simulink model "simulation_ENMPC"  (R2018a)
settings: Solver=ode15s  StartTime=0.0  StopTime=T  RelTol=1e-3
values from neighbouring files (symbols this model uses):
  c = G\Uf    [main_approx_NMPC.m]
  x0 = xk(:)    [find_optimal_NMPC.m]    (also in main_approx_NMPC.m = MPC.Xlb + rand(2,1)*(MPC.Xub - MPC.Xlb))
settings Model: Creator=chakrabarty  LastModifiedBy=chakrabarty
settings OptimizationCC: LifeSpan=inf
settings DebuggingCC: SFExecutionAtInitializationDiag=none
settings HardwareCC: ProdBitPerSizeT=32  ProdBitPerPtrDiffT=32  ProdWordSize=32  ProdHWDeviceType=Specified
settings CodeAppCC: StateflowObjectComments=on

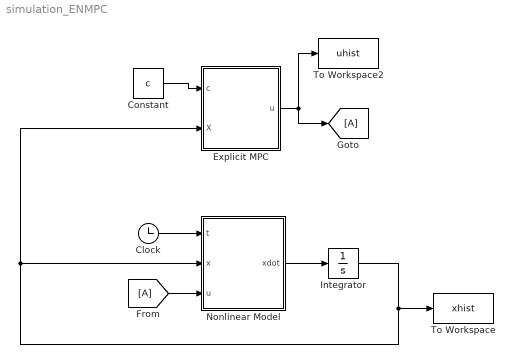
== system simulation_ENMPC ==
  Clock : Clock
  Constant : Constant  Value=c
  Explicit MPC : MATLAB Function  TreatAsAtomicUnit=on
  Integrator : Integrator  InitialCondition=x0
  Nonlinear Model : MATLAB Function  TreatAsAtomicUnit=on
  To Workspace : ToWorkspace  VariableName=xhist  SaveFormat=Timeseries  SampleTime=-1
  To Workspace2 : ToWorkspace  VariableName=uhist  SaveFormat=Timeseries  SampleTime=-1
  wires:
  Constant/1 -> Explicit MPC/1(c)
  Nonlinear Model/1(xdot) -> Integrator/1
  Integrator/1 -> To Workspace/1, Explicit MPC/2(X), Nonlinear Model/2(x)
  Clock/1 -> Nonlinear Model/1(t)
  [A] -> Nonlinear Model/3(u)
  Explicit MPC/1(u) -> [A], To Workspace2/1

== matlab function simulation_ENMPC/Nonlinear Model ==
  data: xdot output; t input; x input; u input
function xdot = fcn(t, x, u)

xdot = [x(2) + u*(0.5 + 0.5*x(1));...
     x(1) + u*(0.5 - 2.0*x(2))];

== matlab function simulation_ENMPC/Explicit MPC ==
  data: u output; c input; X input
function u = fcn(c, X)

% Basis functions
S = @(x,y) [1, x, y, x*y, (2*x^2-1)*y, (2*y^2-1)*x,...
            (4*x^3 - 3*x), (4*y^3 - 3*y)];

% Computing approx NMPC
u = S(X(1), X(2))*c;

% Projection
if u > 2
    u = 2;
end

if u < -2
    u = -2;
end
